simulink model "MatrixWrRd_transpose_SoCB_TopLevel"  (R2020b)
settings: Solver=VariableStepAuto  StartTime=0.0  StopTime=inf  FixedStep=1  RelTol=1e-3  EnableMultiTasking=on
InitFcn:
  | matrix_init();
StopFcn:
  | %hsb_FFT_2D_post;
model workspace (MAT data in the model file):
  hsbmpm = [3707764736; 2; 1; 1; 1; 4]
  mwTaskManagerKernelLatency = 0
  socvcb = containers.Map
  socvcb.serialization.keys = {33.0001220703, 33.0031738281, 34.0001220703, 34.0031738281, 36.0001220703, 36.0008544922, 36.0015869141, 37.0001220703, 37.0008544922, 37.0015869141}
  socvcb.serialization.values : function handle (value not decoded)
  socvcb.serialization.uniformity = 0
  socvcb.serialization.keyType = 'double'
  socvcb.serialization.valueType = 'any'
values from neighbouring files (symbols this model uses):
  MatrixInput = reshape(MatrixInputArr,[N1,N2])    [matrix_init.m]
  N1 = 20    [matrix_init.m]
  N2 = 20    [matrix_init.m]
libraries: simulink x2, hdlsllib x2, socmemlib x2
settings Model: DataTypeOverride=Off  SimulationMode=accelerator  Creator=The MathWorks, Inc.  LastModifiedBy=darenlee
settings SolverCC: PositivePriorityOrder=on
settings DataIOCC: LimitDataPoints=on  SaveFormat=Array  SaveOutput=off  SaveTime=off  ReturnWorkspaceOutputs=off
settings OptimizationCC: BlockReduction=off  ConditionallyExecuteInputs=off  EnhancedBackFolding=on  PassReuseOutputArgsAs=Individual arguments  MaxStackSize=64  OptimizeBlockOrder=speed  DifferentSizesBufferReuse=on  OptimizationCustomize=off  EfficientTunableParamExpr=on
settings DebuggingCC: ReadBeforeWriteMsg=DisableAll  AlgebraicLoopMsg=error  SolverPrmCheckMsg=warning  InheritedTsInSrcMsg=none  MultiTaskCondExecSysMsg=warning  MultiTaskRateTransMsg=warning  IntegerOverflowMsg=none  ParameterPrecisionLossMsg=none  ParameterTunabilityLossMsg=error  AllowSymbolicDim=off  SFUnexpectedBacktrackingDiag=warning  SFNoUnconditionalDefaultTransitionDiag=warning  SFExecutionAtInitializationDiag=none  IntegerSaturationMsg=none  ArithmeticOperatorsInVariantConditions=warning
settings HardwareCC: ProdBitPerLong=64  ProdLargestAtomicInteger=LongLong  ProdLargestAtomicFloat=Double  ProdLongLongMode=on  ProdHWDeviceType=ARM Compatible->ARM 64-bit (LP64)  TargetBitPerPointer=64  TargetBitPerSizeT=64  TargetBitPerPtrDiffT=64  TargetLongLongMode=on  TargetIntDivRoundTo=Zero  TargetEndianess=LittleEndian  TargetWordSize=64  TargetHWDeviceType=Custom Processor->MATLAB Host Computer  ProdEqTarget=off  HardwareBoardFeatureSet=SoCBlockset
settings ModelReferenceCC: PropagateSignalLabelsOutOfModel=off
settings SFSimCC: SimUseLocalCustomCode=off  MATLABDynamicMemAlloc=off  CustomCodeUndefinedFunction=UseInterfaceOnly
settings RTWCC: Description=Embedded Coder  SystemTargetFile=ert.tlc  HardwareBoard=Xilinx Zynq UltraScale+ MPSoC ZCU102 Evaluation Kit  TLCOptions="-aInlineSetEventsForThisBaseRateFcn=TLC_FALSE -aSuppressMultiTaskScheduler=TLC_FALSE  -aRateBasedStepFcn=0"  TemplateMakefile=ert_default_tmf  GenerateReport=on  RTWUseLocalCustomCode=off  Toolchain=Wind River Workbench DIAB 5.9.4.0  IncludeHyperlinkInReport=on  LaunchReport=on  GenerateTraceInfo=on  GenerateTraceReport=on  GenerateTraceReportSl=on  GenerateTraceReportSf=on  GenerateTraceReportEml=on
settings CodeAppCC: ForceParamTrailComments=on  IgnoreCustomStorageClasses=off  OperatorAnnotations=on  SimulinkDataObjDesc=on  SFDataObjDesc=on  InsertBlockDesc=on
settings ConfigComp: CovMetricSettings=dw  CovSaveCumulativeToWorkspaceVar=on  CovSaveSingleToWorkspaceVar=on  CovExternalEMLEnable=off  CovSFcnEnable=off
settings SimscapeCC: SimscapeNormalizeSystem=off

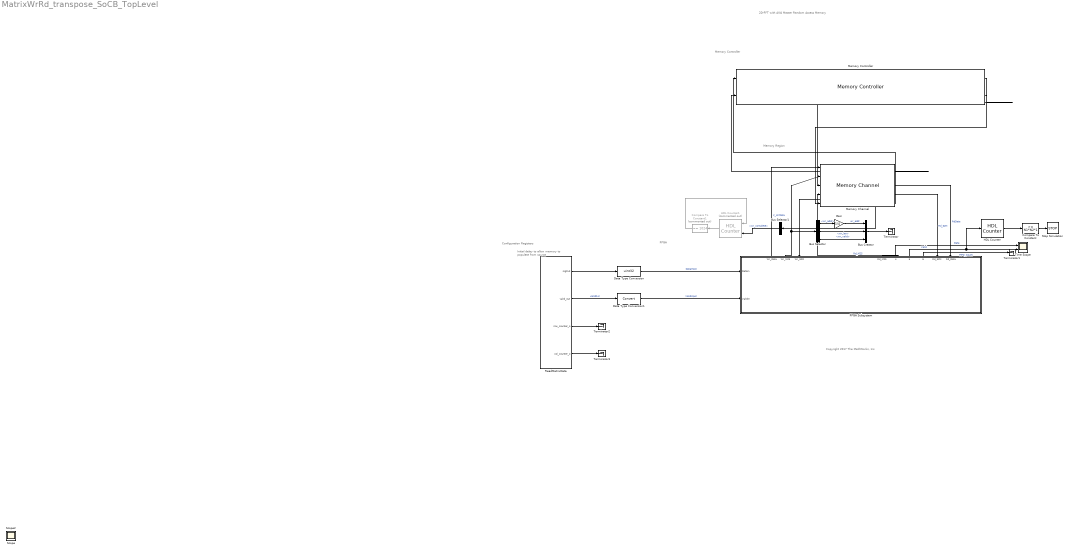
== system MatrixWrRd_transpose_SoCB_TopLevel ==
  note: Initial delay to allow memory
      | to populate from source
  note: Copyright 2017 The MathWorks, Inc.
  note: 2D-FFT with AXI4 Master Random Access Memory
  note: Memory Controller
  note: FPGA
  note: Memory Region
  note: Configuration Registers
  Bus Creator : BusCreator  Inputs=3
  Bus Selector : BusSelector  OutputSignals=wr_addr,wr_len,wr_valid
  Bus Selector1 : BusSelector  OutputSignals=wr_complete
  Compare To Constant : simulink/Logic and Bit Operations/Compare To Constant  relop=>=  const=N1*N2*1  OutDataTypeStr=boolean
  Compare To Constant1 : simulink/Logic and Bit Operations/Compare To Constant  Commented=on  relop===  const=1024  OutDataTypeStr=boolean
  Data Type Conversion : DataTypeConversion  OutDataTypeStr=uint32
  Data Type Conversion1 : DataTypeConversion
  FPGA Subsystem : Subsystem
      settings: PortSchema="{\"entries\":[{\"content\":{\"sides\":[{\"content\":{\"connectorIds\":[\"In4\",\"In5\"]},\"type\":\"ConnectorPlacement.EquallySpacedRectSide\",\"uuid\":\"95616592-d394-44d9-a4ab-e650b479c1a5\"},{\"content\":{\"connectorIds\":[\"Spacer\",\"Spacer\"],\"side\":\"RIGHT\"},\"type\":\"ConnectorPlacement.EquallySpacedRectSide\",\"uuid\":\"c829e787-fd99-46cf-9e25-aac7053e1301\"},{\"content\":{\"connectorIds\":[\"Spacer\",\"Spacer\",\"Out1\",\"Out2\",\"In1\",\"Spacer\",\"Spacer\",\"Spacer\",\"Spacer\",\"Spacer\",\"Out3\",\"Out4\",\"Out5\",\"Out6\",\"In2\",\"In3\",\"Spacer\",\"Spacer\"],\"side\":\"TOP\"},\"type\":\"ConnectorPlacement.EquallySpacedRectSide\",\"uuid\":\"eb1a2cb7-dc8e-4df5-bc07-fca8ee9dc469\"},{\"content\":{\"connectorIds\":[],\"side\":\"BOTTOM\"},\"type\":\"ConnectorPlacement.EquallySpacedRectSide\",\"uuid\":\"03c23e38-125f-4c22-8c5a-d6e512e37bce\"}]},\"type\":\"ConnectorPlacement.EquallySpacedConnector\",\"uuid\":\"e6a43a79-16b9-4956-9439-02e7416ad88d\"}],\"packageUris\":[\"http://schema.mathworks.com/mf0/Connector/19700101\"],\"version\":\"1.0\"}"
  Gain : Gain  Gain=1/4
  HDL Counter : hdlsllib/Sources/HDL Counter  CountType=Free running  CountInit=0  CountStep=1  CountMax=25  CountFromType=Initial value  CountFrom=0  CountResetPort=off  CountLoadPort=off  CountEnbPort=on  CountDirPort=off  CountDataType=Unsigned  CountWordLen=32  CountFracLen=0  CountSampTime=1
  HDL Counter1 : hdlsllib/Sources/HDL Counter  Commented=on  CountType=Free running  CountInit=0  CountStep=1  CountMax=25  CountFromType=Initial value  CountFrom=0  CountResetPort=on  CountLoadPort=off  CountEnbPort=on  CountDirPort=off  CountDataType=Unsigned  CountWordLen=32  CountFracLen=0  CountSampTime=1
  Memory Channel : socmemlib/Memory Channel  InstantiateOnLoad=on  ChannelType=AXI4 Random Access  MRBufferSize=8192*40*4*2  MRNumBuffers=1  BurstLengthWriterChIf=1024  BurstLengthReaderChIf=1024  UseValuesFromTargetHardwareResources=on  ReaderWriterUseSameValues=on  FIFODepthWriter=8  FIFODepthReader=8  FIFOAFullDepthWriter=6  FIFOAFullDepthReader=6  ICClockFrequencyWriter=300  ICClockFrequencyReader=300  ICDataWidthWriter=32  ICDataWidthReader=32  ChDimensionsWriterChIf=1  ChTypeWriterChIf=uint32  ChFrameSampleTimeWriterChIf=1  OutSigSpecMatchesInSigSpec=off  ChDimensionsReaderChIf=1  ChTypeWithInhReaderChIf=Inherit: Same as input  ChFrameSampleTimeReaderChIf=1  InsertInactivePixelClocksReaderChIf=off  FrameSizeReaderChIf=160x120p  ProtocolWriter=AXI4  ProtocolReader=AXI4  ChTypeReaderChIf=uint32  LastTargetBoard=Xilinx Zynq UltraScale+ MPSoC ZCU102 Evaluation Kit  Beta2Compatible=off  MRRegionSize=2621440  DiagnosticLevel=No debug  MRBaseAddress=hex2dec('00010000')  UseTargetGlobalValues=off  InterruptHandlingTimeWriterChIf=10e-6  BufferEventIDWriterChIf=NOT_USED  BufferLengthReaderChIf=NOT_USED  InterruptHandlingTimeReaderChIf=10e-6  BufferEventIDReaderChIf=NOT_USED
      settings: SourceProductBaseCode=HW
  Memory Controller : socmemlib/Memory Controller  InstantiateOnLoad=on  NumMasters=2  ICArbitrationPolicy=Round robin  UseValuesFromTargetHardwareResources=on  ControllerFrequency=300  ControllerDataWidth=128  BandwidthDerating=2.3  WriteFirstTransferLatency=4  ReadFirstTransferLatency=5  WriteLastTransferLatency=4  ReadLastTransferLatency=1  LastTargetBoard=Xilinx Zynq UltraScale+ MPSoC ZCU102 Evaluation Kit  DiagnosticLevel=No debug  MAX_NUM_MASTERS=12  DDRRefreshLength=4  DDRRefreshInterval=7.8  PlotTimeResolution=100e-6
      settings: SourceProductName=HDL System Blockset
  ReadMatrixData : MATLAB Function  TreatAsAtomicUnit=on  SystemSampleTime=Ts  mask{MatrixInput=MatrixInput, ValidGap=N1*(16-1), Ts=1}
      mask prompts: MatrixInput "Matrix value"; ValidGap "Valid Gap between columns"; Ts "Sample Time"
  Stop Simulation : Stop
  Terminator{,1..3} (4 alike) : Terminator
  Time Scope : Scope  NumInputPorts=2
  Scope : Scope
  Scope2 : Scope
  wires:
  FPGA Subsystem/1(Wr_Data) -> Memory Channel/1  "ir_WrData"
  FPGA Subsystem/2(Wr_M2S) -> Memory Channel/2, Bus Selector/1
  Memory Channel/1 -> Bus Selector1/1, FPGA Subsystem/1(Wr_S2M)
  Memory Channel/2 -> Memory Controller/1
  Memory Controller/1 -> Memory Channel/3
  Memory Channel/5 -> Memory Controller/2
  Memory Controller/2 -> Memory Channel/5
  FPGA Subsystem/3(Rd_M2S) -> Memory Channel/4  "Rd_M2S"
  Memory Channel/4 -> FPGA Subsystem/2(Rd_S2M)  "Rd_S2M"
  Memory Channel/3 -> FPGA Subsystem/3(Rd_Data)  "RdData"
  ReadMatrixData/1(sigOut) -> Data Type Conversion/1
  Data Type Conversion/1 -> FPGA Subsystem/4(DataIn)  "DataInput"
  Data Type Conversion1/1 -> FPGA Subsystem/5(ValidIn)  "ValidInput"
  ReadMatrixData/2(valid_out) -> Data Type Conversion1/1  "validOut"
  ReadMatrixData/3(row_counter_o) -> Terminator2/1
  ReadMatrixData/4(col_counter_o) -> Terminator3/1
  FPGA Subsystem/4(matrix_rd_out) -> Time Scope/1  "Data"
  FPGA Subsystem/5(matrix_rd_valid) -> HDL Counter/1, Time Scope/2  "Valid"
  Bus Selector/1 -> Gain/1  "<wr_addr>"
  Gain/1 -> Bus Creator/1  "wr_addr"
  Bus Selector/2 -> Bus Creator/2  "<wr_len>"
  Bus Selector/3 -> Bus Creator/3  "<wr_valid>"
  Bus Creator/1 -> Terminator/1
  HDL Counter/1 -> Compare To Constant/1
  Compare To Constant/1 -> Stop Simulation/1
  FPGA Subsystem/6(FIFO_Count) -> Terminator1/1  "FIFO_Count"
  Bus Selector1/1 -> HDL Counter1/2  "<wr_complete>"
  HDL Counter1/1 -> Compare To Constant1/1
  Compare To Constant1/1 -> HDL Counter1/1

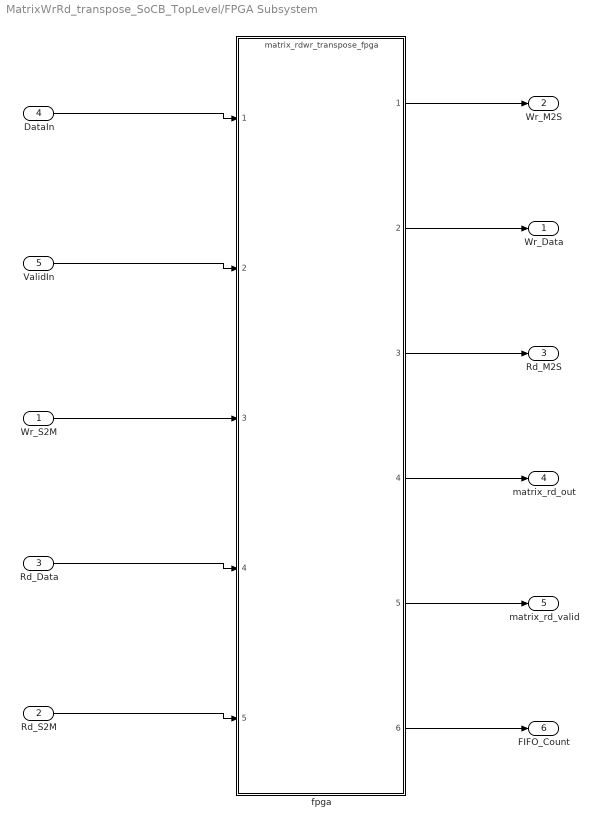
== system MatrixWrRd_transpose_SoCB_TopLevel/FPGA Subsystem ==
  Wr_S2M : Inport
  Rd_S2M : Inport  Port=2
  Rd_Data : Inport  Port=3
  DataIn : Inport  Port=4
  ValidIn : Inport  Port=5
  fpga : ModelReference  ModelNameDialog=matrix_rdwr_transpose_fpga.slx  SimulationMode=Normal  ModelReferenceVersion=3.0
  Wr_Data : Outport  SampleTime=1  VectorParamsAs1DForOutWhenUnconnected=off
  Wr_M2S : Outport  Port=2  SampleTime=1  VectorParamsAs1DForOutWhenUnconnected=off
  Rd_M2S : Outport  Port=3  SampleTime=1  VectorParamsAs1DForOutWhenUnconnected=off
  matrix_rd_out : Outport  Port=4
  matrix_rd_valid : Outport  Port=5
  FIFO_Count : Outport  Port=6
  wires:
  fpga/2 -> Wr_Data/1
  fpga/1 -> Wr_M2S/1
  fpga/3 -> Rd_M2S/1
  DataIn/1 -> fpga/1
  ValidIn/1 -> fpga/2
  Wr_S2M/1 -> fpga/3
  Rd_S2M/1 -> fpga/5
  Rd_Data/1 -> fpga/4
  fpga/4 -> matrix_rd_out/1
  fpga/5 -> matrix_rd_valid/1
  fpga/6 -> FIFO_Count/1

== matlab function MatrixWrRd_transpose_SoCB_TopLevel/ReadMatrixData ==
  data: sigOut output; valid_out output; MatrixInput parameter; row_counter_o output; col_counter_o output; ValidGap parameter
function [sigOut,valid_out,row_counter_o,col_counter_o] = fcn(MatrixInput,ValidGap)
    persistent row_counter col_counter stop_write;
%     ValidGap = 10;
    if isempty(row_counter)
        row_counter = uint32(1);
        col_counter = uint32(1);
        stop_write = false;
      
    end
    [n_rows,m_cols] = size(MatrixInput);
    max_row_count = n_rows + ValidGap;

    %% Read value from matrix
    if row_counter <= n_rows && ~stop_write
        sigOut = MatrixInput(row_counter,col_counter);
        valid_out = true;
    else
        sigOut = 0; % insert valid gap 
        valid_out = false;
    end
    
    row_counter_o = row_counter;
    col_counter_o = col_counter;
    
    %% Update counters
    if row_counter < max_row_count 
        row_counter(:) = row_counter + 1; 
    else
        row_counter(:) = 1;
        if col_counter < m_cols
            col_counter(:) = col_counter + 1; % next column
        else
            col_counter(:) = 1; % reset to beginning of matrix
            stop_write = false;
        end
    end

end
